simulink model "sampleModel1441"  (R2023a)
settings: Solver=VariableStepAuto  StartTime=0.0  StopTime=10.0  RelTol=1e-3
libraries: hdlsllib x3
settings Model: Creator=user1  LastModifiedBy=user1

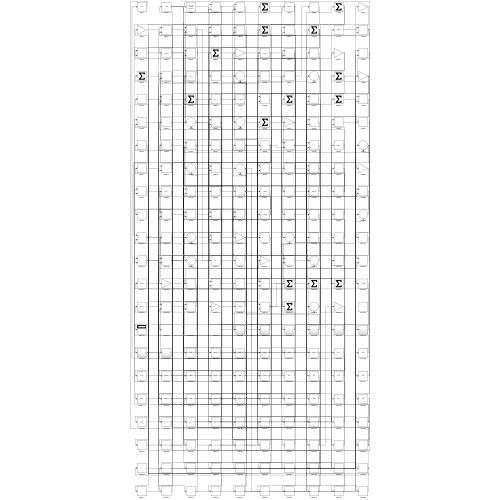
[thumbnail: Simulink's stored preview of the top-level diagram]
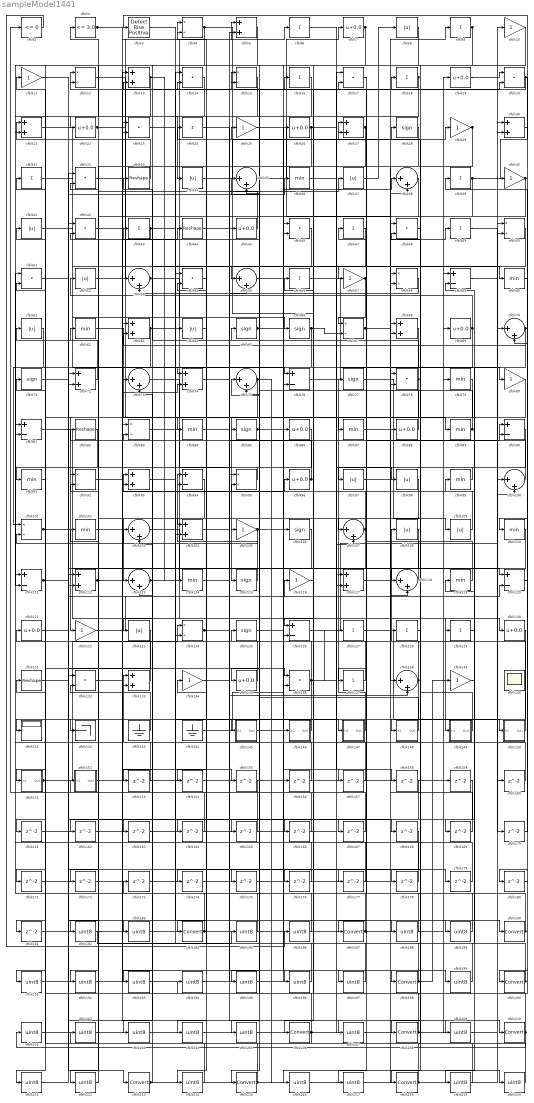
== system sampleModel1441 ==
  cfblk1 : hdlsllib/Logic and Bit Operations/Compare To Zero  relop=<=  OutDataTypeStr=boolean
  cfblk{10..11,25,29,40,57,80,105,116,122,134,139} (12 alike) : Gain
  cfblk{35,38,53,55,70,73,75,100,103,107,113,118,138} (13 alike) : Sum  Inputs=|++
  cfblk{4,12,15,50,58,67,83,92,95,101,124} (11 alike) : Product  Inputs=*/  RndMeth=Zero  SaturateOnIntegerOverflow=on
  cfblk{36,60,62,79,84,87,89,91,99,102,110,114,119} (13 alike) : MinMax
  cfblk{5,13,21,27,30,63,68,72,74,93,104,112,117,133} (14 alike) : Sum
  cfblk{28,65..66,71,77,85,106,115,125} (9 alike) : Signum
  cfblk{8,34,37,41,52,61,64,97..98,108..109,123} (12 alike) : Abs  SaturateOnIntegerOverflow=off
  cfblk{59,76,81,90,94,111,120,126} (8 alike) : Sum  Inputs=+-
  cfblk{7,19,22,26,45,69,86,88,96,121,130,135} (12 alike) : Bias  Bias=0.0  SaturateOnIntegerOverflow=off
  cfblk{6,9,16,18,24,31,39,43,47,49,56,127..129,137} (15 alike) : Sum  Inputs=+
  cfblk{33,44,82,131} (4 alike) : Reshape
  cfblk{14,17,20,23,32,42,46,48,51,54,78,132,136} (13 alike) : DotProduct  OutDataTypeStr=Inherit: Inherit via internal rule
  cfblk140 : Scope
      settings: Floating=on
  cfblk141 : Display
  cfblk142 : Terminator
  cfblk143 : Ground
  cfblk144 : Ground
  cfblk145 : Subsystem
      settings: LibrarySourceBlock=|
      | hdlsllib/Ports &
      | Subsystems/Subsystem
  cfblk146 : Subsystem
      settings: LibrarySourceBlock=|
      | hdlsllib/Ports &
      | Subsystems/Subsystem
  cfblk147 : Subsystem
      settings: LibrarySourceBlock=|
      | hdlsllib/Ports &
      | Subsystems/Subsystem
  cfblk148 : Subsystem
      settings: LibrarySourceBlock=|
      | hdlsllib/Ports &
      | Subsystems/Subsystem
  cfblk149 : Subsystem
      settings: LibrarySourceBlock=|
      | hdlsllib/Ports &
      | Subsystems/Subsystem
  cfblk150 : Subsystem
      settings: LibrarySourceBlock=|
      | hdlsllib/Ports &
      | Subsystems/Subsystem
  cfblk151 : Subsystem
      settings: LibrarySourceBlock=|
      | hdlsllib/Ports &
      | Subsystems/Subsystem
  cfblk152 : Subsystem
      settings: LibrarySourceBlock=|
      | hdlsllib/Ports &
      | Subsystems/Subsystem
  cfblk{153..181} (29 alike) : Delay  SampleTime=1
  cfblk{182..183,185..186,188..189,191..197,199,201..205,207,209,211..212,214,216..217,219..220} (28 alike) : DataTypeConversion  OutDataTypeStr=uint8  SaturateOnIntegerOverflow=off  RndMeth=Floor
  cfblk{184,187,190,198,200,206,208,210,213,215,218} (11 alike) : DataTypeConversion  SaturateOnIntegerOverflow=off  RndMeth=Floor
  cfblk2 : hdlsllib/Logic and Bit Operations/Compare To Constant  relop=<=  const=3.0  OutDataTypeStr=boolean
  cfblk3 : hdlsllib/Logic and Bit Operations/Detect Rise Positive  vinit=0  OutDataTypeStr=boolean
  wires:
  cfblk76/1 -> cfblk80/1
  cfblk94/1 -> cfblk113/1
  cfblk120/1 -> cfblk39/1
  cfblk77/1 -> cfblk109/1
  cfblk70/1 -> cfblk63/2, cfblk219/1
  cfblk147/1(Out1) -> cfblk77/1
  cfblk151/1(Out1) -> cfblk124/1, cfblk116/1
  cfblk130/1 -> cfblk133/1
  cfblk31/1 -> cfblk66/1
  cfblk35/1 -> cfblk7/1
  cfblk62/1 -> cfblk115/1
  cfblk150/1(Out1) -> cfblk108/1
  cfblk99/1 -> cfblk97/1
  cfblk4/1 -> cfblk135/1, cfblk22/1
  cfblk75/1 -> cfblk156/1, cfblk191/1, cfblk205/1
  cfblk54/1 -> cfblk184/1
  cfblk117/1 -> cfblk58/2
  cfblk52/1 -> cfblk5/1
  cfblk12/1 -> cfblk85/1
  cfblk152/1(Out1) -> cfblk59/1
  cfblk69/1 -> cfblk107/1, cfblk52/1
  cfblk6/1 -> cfblk98/1
  cfblk126/1 -> cfblk70/1
  cfblk81/1 -> cfblk118/1
  cfblk105/1 -> cfblk101/2, cfblk38/1, cfblk216/1
  cfblk37/1 -> cfblk8/1
  cfblk127/1 -> cfblk150/1(In1)
  cfblk11/1 -> cfblk213/1
  cfblk113/1 -> cfblk6/1, cfblk163/1
  cfblk34/1 -> cfblk29/1
  cfblk33/1 -> cfblk21/1
  cfblk78/1 -> cfblk122/1, cfblk33/1
  cfblk103/1 -> cfblk130/1
  cfblk63/1 -> cfblk18/1, cfblk111/2
  cfblk115/1 -> cfblk94/1
  cfblk8/1 -> cfblk126/1
  cfblk129/1 -> cfblk59/2
  cfblk20/1 -> cfblk14/2, cfblk180/1
  cfblk23/1 -> cfblk190/1
  cfblk56/1 -> cfblk128/1
  cfblk39/1 -> cfblk3/1, cfblk212/1
  cfblk40/1 -> cfblk76/1, cfblk93/2
  cfblk116/1 -> cfblk16/1
  cfblk25/1 -> cfblk138/1
  cfblk97/1 -> cfblk88/1
  cfblk83/1 -> cfblk105/1
  cfblk95/1 -> cfblk92/1
  cfblk18/1 -> cfblk21/2, cfblk13/2, cfblk174/1
  cfblk74/1 -> cfblk37/1
  cfblk114/1 -> cfblk138/2
  cfblk137/1 -> cfblk41/1
  cfblk41/1 -> cfblk60/1
  cfblk93/1 -> cfblk64/1
  cfblk10/1 -> cfblk208/1
  cfblk118/1 -> cfblk12/1
  cfblk144/1 -> cfblk26/1
  cfblk15/1 -> cfblk34/1
  cfblk146/1(Out1) -> cfblk141/1
  cfblk72/1 -> cfblk31/1
  cfblk131/1 -> cfblk136/1
  cfblk59/1 -> cfblk100/2
  cfblk9/1 -> cfblk75/2, cfblk126/2
  cfblk47/1 -> cfblk84/1
  cfblk53/1 -> cfblk146/1(In1), cfblk147/1(In1)
  cfblk148/1(Out1) -> cfblk95/2
  cfblk111/1 -> cfblk179/1, cfblk209/1
  cfblk132/1 -> cfblk210/1
  cfblk66/1 -> cfblk67/2, cfblk153/1, cfblk192/1
  cfblk2/1 -> cfblk89/1, cfblk4/2, cfblk136/2
  cfblk119/1 -> cfblk93/1
  cfblk19/1 -> cfblk20/1
  cfblk27/1 -> cfblk103/2, cfblk166/1
  cfblk5/1 -> cfblk91/1
  cfblk21/1 -> cfblk86/1
  cfblk143/1 -> cfblk62/1
  cfblk45/1 -> cfblk2/1
  cfblk149/1(Out1) -> cfblk24/1
  cfblk16/1 -> cfblk104/1
  cfblk61/1 -> cfblk101/1
  cfblk104/1 -> cfblk90/1
  cfblk67/1 -> cfblk9/1, cfblk20/2
  cfblk68/1 -> cfblk215/1
  cfblk51/1 -> cfblk72/2
  cfblk122/1 -> cfblk40/1
  cfblk107/1 -> cfblk15/1, cfblk112/2
  cfblk57/1 -> cfblk27/1, cfblk67/1
  cfblk109/1 -> cfblk83/2
  cfblk73/1 -> cfblk87/1
  cfblk7/1 -> cfblk81/2, cfblk73/1
  cfblk135/1 -> cfblk94/2
  cfblk145/1(Out1) -> cfblk28/1
  cfblk65/1 -> cfblk129/1, cfblk195/1, cfblk197/1
  cfblk133/1 -> cfblk71/1
  cfblk48/1 -> cfblk218/1
  cfblk79/1 -> cfblk206/1
  cfblk58/1 -> cfblk53/2
  cfblk60/1 -> cfblk110/1
  cfblk80/1 -> cfblk148/1(In1)
  cfblk22/1 -> cfblk55/1, cfblk164/1
  cfblk90/1 -> cfblk137/1
  cfblk38/1 -> cfblk74/1
  cfblk30/1 -> cfblk200/1
  cfblk17/1 -> cfblk187/1
  cfblk134/1 -> cfblk198/1
  cfblk112/1 -> cfblk96/1, cfblk15/2, cfblk74/2
  cfblk136/1 -> cfblk90/2, cfblk127/1, cfblk32/2, cfblk175/1
  cfblk85/1 -> cfblk106/1, cfblk188/1
  cfblk106/1 -> cfblk133/2
  cfblk24/1 -> cfblk55/2
  cfblk28/1 -> cfblk142/1
  cfblk88/1 -> cfblk47/1
  cfblk89/1 -> cfblk35/2, cfblk43/1
  cfblk29/1 -> cfblk78/2, cfblk57/1
  cfblk92/1 -> cfblk44/1
  cfblk138/1 -> cfblk103/1, cfblk214/1
  cfblk96/1 -> cfblk82/1, cfblk25/1
  cfblk124/1 -> cfblk4/1, cfblk120/2
  cfblk101/1 -> cfblk149/1(In1), cfblk36/1
  cfblk13/1 -> cfblk151/1(In1), cfblk114/1
  cfblk100/1 -> cfblk27/2
  cfblk14/1 -> cfblk123/1
  cfblk26/1 -> cfblk120/1, cfblk104/2
  cfblk87/1 -> cfblk49/1
  cfblk43/1 -> cfblk145/1(In1), cfblk42/2
  cfblk153/1 -> cfblk72/1
  cfblk64/1 -> cfblk154/1
  cfblk154/1 -> cfblk118/2
  cfblk42/1 -> cfblk155/1
  cfblk155/1 -> cfblk1/1
  cfblk156/1 -> cfblk81/1
  cfblk55/1 -> cfblk157/1
  cfblk157/1 -> cfblk35/1
  cfblk36/1 -> cfblk158/1
  cfblk160/1 -> cfblk92/2
  cfblk86/1 -> cfblk161/1
  cfblk161/1 -> cfblk117/2
  cfblk98/1 -> cfblk162/1
  cfblk163/1 -> cfblk124/2
  cfblk164/1 -> cfblk51/2
  cfblk3/1 -> cfblk165/1
  cfblk165/1 -> cfblk13/1
  cfblk166/1 -> cfblk63/1
  cfblk71/1 -> cfblk167/1
  cfblk167/1 -> cfblk83/1
  cfblk125/1 -> cfblk168/1
  cfblk139/1 -> cfblk169/1
  cfblk169/1 -> cfblk58/1
  cfblk49/1 -> cfblk170/1
  cfblk170/1 -> cfblk70/2
  cfblk123/1 -> cfblk171/1
  cfblk171/1 -> cfblk95/1
  cfblk110/1 -> cfblk172/1
  cfblk172/1 -> cfblk53/1
  cfblk173/1 -> cfblk38/2
  cfblk174/1 -> cfblk76/2
  cfblk175/1 -> cfblk107/2
  cfblk108/1 -> cfblk176/1
  cfblk176/1 -> cfblk111/1
  cfblk32/1 -> cfblk177/1
  cfblk177/1 -> cfblk75/1
  cfblk128/1 -> cfblk178/1
  cfblk178/1 -> cfblk78/1
  cfblk179/1 -> cfblk12/2
  cfblk91/1 -> cfblk181/1
  cfblk181/1 -> cfblk5/2
  cfblk159/1 -> cfblk182/1
  cfblk121/1 -> cfblk183/1
  cfblk183/1 -> cfblk159/1
  cfblk184/1 -> cfblk112/1, cfblk69/1
  cfblk182/1 -> cfblk185/1
  cfblk185/1 -> cfblk54/1
  cfblk1/1 -> cfblk186/1
  cfblk186/1 -> cfblk54/2
  cfblk187/1 -> cfblk32/1, cfblk51/1
  cfblk188/1 -> cfblk17/1
  cfblk162/1 -> cfblk189/1
  cfblk189/1 -> cfblk17/2
  cfblk190/1 -> cfblk42/1, cfblk119/1
  cfblk191/1 -> cfblk23/1
  cfblk192/1 -> cfblk23/2
  cfblk46/1 -> cfblk193/1
  cfblk193/1 -> cfblk45/1
  cfblk180/1 -> cfblk194/1
  cfblk194/1 -> cfblk46/1
  cfblk195/1 -> cfblk46/2
  cfblk102/1 -> cfblk196/1
  cfblk196/1 -> cfblk113/2
  cfblk197/1 -> cfblk102/1
  cfblk198/1 -> cfblk73/2, cfblk139/1, cfblk125/1
  cfblk84/1 -> cfblk199/1
  cfblk199/1 -> cfblk134/1
  cfblk200/1 -> cfblk14/1, cfblk99/1
  cfblk201/1 -> cfblk30/1
  cfblk202/1 -> cfblk30/2
  cfblk50/1 -> cfblk203/1
  cfblk203/1 -> cfblk117/1
  cfblk168/1 -> cfblk204/1
  cfblk204/1 -> cfblk50/1
  cfblk205/1 -> cfblk50/2
  cfblk206/1 -> cfblk202/1, cfblk19/1, cfblk65/1
  cfblk44/1 -> cfblk207/1
  cfblk207/1 -> cfblk79/1
  cfblk208/1 -> cfblk56/1, cfblk131/1
  cfblk209/1 -> cfblk10/1
  cfblk210/1 -> cfblk201/1, cfblk152/1(In1)
  cfblk82/1 -> cfblk211/1
  cfblk211/1 -> cfblk132/1
  cfblk212/1 -> cfblk132/2
  cfblk213/1 -> cfblk173/1, cfblk100/1
  cfblk214/1 -> cfblk11/1
  cfblk215/1 -> cfblk61/1, cfblk220/1
  cfblk216/1 -> cfblk68/1
  cfblk158/1 -> cfblk217/1
  cfblk217/1 -> cfblk68/2
  cfblk218/1 -> cfblk160/1, cfblk121/1
  cfblk219/1 -> cfblk48/1
  cfblk220/1 -> cfblk48/2

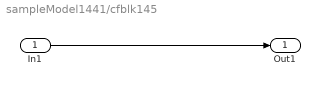
== system sampleModel1441/cfblk145 ==
  In1 : Inport
  Out1 : Outport
  wires:
  In1/1 -> Out1/1

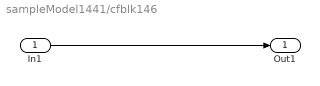
== system sampleModel1441/cfblk146 ==
  In1 : Inport
  Out1 : Outport
  wires:
  In1/1 -> Out1/1

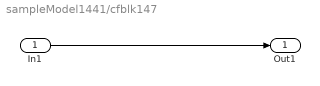
== system sampleModel1441/cfblk147 ==
  In1 : Inport
  Out1 : Outport
  wires:
  In1/1 -> Out1/1

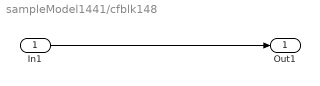
== system sampleModel1441/cfblk148 ==
  In1 : Inport
  Out1 : Outport
  wires:
  In1/1 -> Out1/1

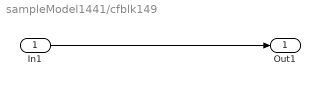
== system sampleModel1441/cfblk149 ==
  In1 : Inport
  Out1 : Outport
  wires:
  In1/1 -> Out1/1

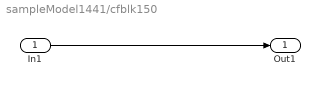
== system sampleModel1441/cfblk150 ==
  In1 : Inport
  Out1 : Outport
  wires:
  In1/1 -> Out1/1

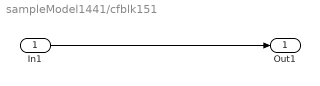
== system sampleModel1441/cfblk151 ==
  In1 : Inport
  Out1 : Outport
  wires:
  In1/1 -> Out1/1

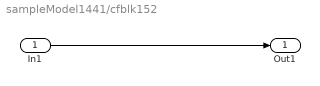
== system sampleModel1441/cfblk152 ==
  In1 : Inport
  Out1 : Outport
  wires:
  In1/1 -> Out1/1
